simulink model "fec_top_multiple_clk_domains_tb"  (R2023b)
settings: Solver=FixedStepDiscrete  StartTime=0.0  StopTime=10.0  RelTol=1e-3
undefined symbols (not defined in the file or in its folder): fec_clk, rs_clk
settings Model: DataTypeOverride=Off  Creator=foregan  LastModifiedBy=foregan
settings OptimizationCC: BlockReduction=off  ConditionallyExecuteInputs=off  DefaultParameterBehavior=Inlined  InheritOutputTypeSmallerThanSingle=on
settings DebuggingCC: AlgebraicLoopMsg=error  SingleTaskRateTransMsg=error
settings HardwareCC: ProdBitPerPointer=32  ProdBitPerSizeT=32  ProdBitPerPtrDiffT=32  ProdLargestAtomicFloat=None  ProdIntDivRoundTo=Undefined  ProdEndianess=Unspecified  ProdWordSize=32  ProdHWDeviceType=ASIC/FPGA->ASIC/FPGA  TargetBitPerPointer=64  TargetBitPerSizeT=64  TargetBitPerPtrDiffT=64  TargetLongLongMode=on  TargetIntDivRoundTo=Zero  TargetEndianess=LittleEndian  TargetWordSize=64  TargetHWDeviceType=Custom Processor->MATLAB Host Computer  ProdEqTarget=off

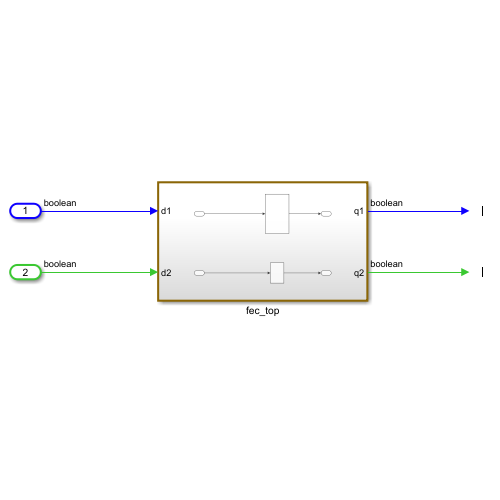
[thumbnail: Simulink's stored preview of the top-level diagram]
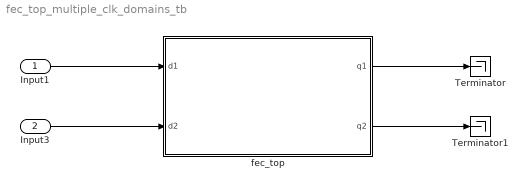
== system fec_top_multiple_clk_domains_tb ==
  Input1 : Inport  OutDataTypeStr=boolean  SampleTime=1/rs_clk
  Input3 : Inport  Port=2  OutDataTypeStr=boolean  SampleTime=1/fec_clk
  Terminator : Terminator
  Terminator1 : Terminator
  fec_top : Subsystem
  wires:
  Input3/1 -> fec_top/2(d2)
  Input1/1 -> fec_top/1(d1)
  fec_top/1(q1) -> Terminator/1
  fec_top/2(q2) -> Terminator1/1

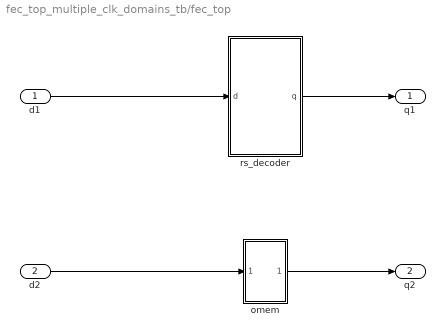
== system fec_top_multiple_clk_domains_tb/fec_top ==
  d1 : Inport
  d2 : Inport  Port=2
  omem : Subsystem
  rs_decoder : Subsystem
  q1 : Outport
  q2 : Outport  Port=2
  wires:
  rs_decoder/1(q) -> q1/1
  d2/1 -> omem/1(In1)
  omem/1(Out1) -> q2/1
  d1/1 -> rs_decoder/1(d)

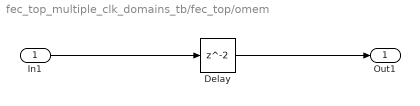
== system fec_top_multiple_clk_domains_tb/fec_top/omem ==
  In1 : Inport
  Delay : Delay
  Out1 : Outport
  wires:
  Delay/1 -> Out1/1
  In1/1 -> Delay/1

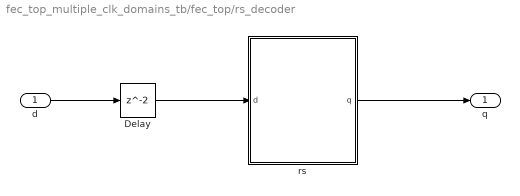
== system fec_top_multiple_clk_domains_tb/fec_top/rs_decoder ==
  d : Inport
  Delay : Delay
  rs : Subsystem
  q : Outport
  wires:
  rs/1(q) -> q/1
  Delay/1 -> rs/1(d)
  d/1 -> Delay/1

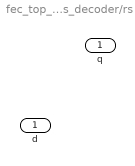
== system fec_top_multiple_clk_domains_tb/fec_top/rs_decoder/rs ==
  d : Inport  OutDataTypeStr=boolean
  q : Outport  OutDataTypeStr=boolean  SampleTime=1/rs_clk
